simulink model "sgm_iox_io397_digital_loopback"  (R2020b)
settings: Solver=FixedStepDiscrete  StartTime=0.0  StopTime=inf  FixedStep=0.001  RelTol=1e-3  EnableMultiTasking=on
undefined symbols (not defined in the file): IO397
libraries: speedgoatlib_fpga_dio x2, speedgoatlib_fpga x1
settings Model: SimulationMode=external  ExtModeArmWhenConnect=off  Creator=ylee  LastModifiedBy=daniel.fonte
settings SolverCC: ConcurrentTasks=on  PositivePriorityOrder=on  AutoInsertRateTranBlk=on  InsertRTBMode=Never (minimum delay)
settings DataIOCC: SaveFormat=Array  SignalLoggingSaveFormat=ModelDataLogs  SaveState=on
settings OptimizationCC: BlockReduction=off  OptimizeBlockIOStorage=off  BufferReuse=off  GlobalBufferReuse=off  ExpressionFolding=off  ExpressionDepthLimit=2147483647  LocalBlockOutputs=off  InitFltsAndDblsToZero=on  OptimizeDataStoreBuffers=off  BusAssignmentInplaceUpdate=off
settings DebuggingCC: UnderspecifiedInitializationDetection=Classic  MergeDetectMultiDrivingBlocksExec=none  SolverPrmCheckMsg=warning  FcnCallInpInsideContextMsg=warning  AllowSymbolicDim=off  StateNameClashWarn=warning  SFUnexpectedBacktrackingDiag=warning  SFNoUnconditionalDefaultTransitionDiag=warning  SFExecutionAtInitializationDiag=none  ArithmeticOperatorsInVariantConditions=warning
settings HardwareCC: ProdBitPerLong=64  ProdLongLongMode=on  ProdHWDeviceType=Intel->x86-64 (Linux 64)
settings ModelReferenceCC: PropagateSignalLabelsOutOfModel=off
settings SFSimCC: SimCustomHeaderCode="#include \"my_type.h\""  SimUseLocalCustomCode=off  SimParseCustomCode=off  CustomCodeUndefinedFunction=UseInterfaceOnly
settings RTWCC: Description=Simulink Real-Time  SystemTargetFile=slrealtime.tlc  TemplateMakefile=slrealtime_default_tmf  RTWUseLocalCustomCode=off  Toolchain=Simulink Real-Time Toolchain  BuildConfiguration=Faster Runs  CodeExecutionProfiling=on  TargetLang=C++
settings CodeAppCC: StateflowObjectComments=on
settings ConfigComp: CovMetricSettings=dw  CovSaveCumulativeToWorkspaceVar=on  CovSaveSingleToWorkspaceVar=on  CovExternalEMLEnable=off  CovSFcnEnable=off

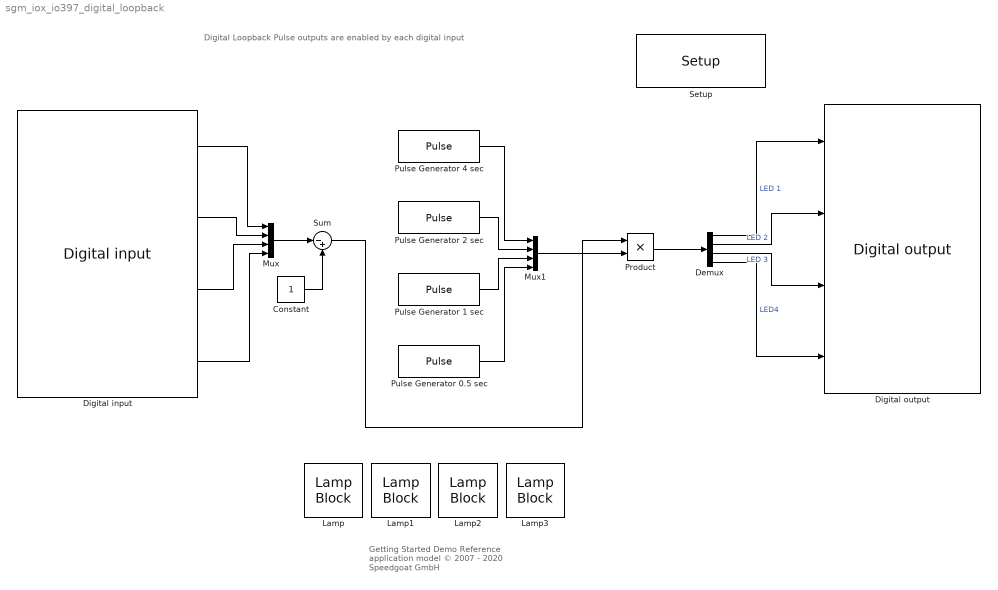
== system sgm_iox_io397_digital_loopback ==
  note: Digital Loopback
      | Pulse outputs are enabled by each digital input
  note: Getting Started Demo
      | Reference application model
      | © 2007 - 2020 Speedgoat GmbH
  Constant : Constant
  Demux : Demux
  Digital input : speedgoatlib_fpga_dio/Digital input  id=1  chan=[1 2 3 4]  ts=0.001  pciSlot=-1  board=IO397-50k  vectorizeOutput=off
      settings: SourceProductName=Simulink Real-Time: Speedgoat I/O Driver Library
  Digital output : speedgoatlib_fpga_dio/Digital output  id=1  chan=[5 6 7 8]  init=[0]  reset=[0]  vectorizeInput=off  ts=0.001  pciSlot=-1  board=IO397-50k
      settings: SourceProductName=Simulink Real-Time: Speedgoat I/O Driver Library
  Lamp{,1..3} (4 alike) : LampBlock
  Mux : Mux
  Mux1 : Mux
  Product : Product
  Pulse Generator 0.5 sec : DiscretePulseGenerator  PulseType=Time based  Period=0.5  PulseWidth=50
  Pulse Generator 1 sec : DiscretePulseGenerator  PulseType=Time based  Period=1  PulseWidth=50
  Pulse Generator 2 sec : DiscretePulseGenerator  PulseType=Time based  PulseWidth=50
  Pulse Generator 4 sec : DiscretePulseGenerator  PulseType=Time based  Period=4  PulseWidth=50
  Setup : speedgoatlib_fpga/Setup/Setup  board=IO397-50k  id=1  device_id=1  frontIO=None  rearIO=None  bitstreamFile=speedgoat_IO397_50k_CI_IO397_DUT_DEMO  rev=1.0  timestamp_string=05/10/17 09:15:16  fpgaFreq=75 MHz  fpgaTick=13.33 ns  ProgSpiFlash=off  ProgBPIFlash=off  pciSlot=-1  PullRPort0=pull-up 3.3V  VioPort0=3.3V  PullRPort1=pull-up 3.3V  VioPort1=3.3V  PullRPort2=pull-up 3.3V  VioPort2=3.3V  PullRPort3=pull-up 3.3V  VioPort3=3.3V  PullRPort4=pull-up 3.3V  VioPort4=3.3V  PullRPort5=pull-up 3.3V  VioPort5=3.3V  PullRPort6=pull-up 3.3V  VioPort6=3.3V  PullRPort15=pull-up 3.3V  PullRPort31=pull-up 3.3V  PullRPort47=pull-up 3.3V  PullRPort63=pull-up 3.3V
      settings: SourceProductName=Simulink Real-Time: Speedgoat I/O Driver Library
  Sum : Sum  Inputs=|-+
  wires:
  Digital input/2 -> Mux/2
  Digital input/3 -> Mux/3
  Digital input/1 -> Mux/1
  Digital input/4 -> Mux/4
  Pulse Generator 2 sec/1 -> Mux1/2
  Pulse Generator 1 sec/1 -> Mux1/3
  Pulse Generator 4 sec/1 -> Mux1/1
  Pulse Generator 0.5 sec/1 -> Mux1/4
  Mux/1 -> Sum/1
  Constant/1 -> Sum/2
  Sum/1 -> Product/1
  Mux1/1 -> Product/2
  Product/1 -> Demux/1
  Demux/2 -> Digital output/2  "LED 2"
  Demux/3 -> Digital output/3  "LED 3"
  Demux/1 -> Digital output/1  "LED 1"
  Demux/4 -> Digital output/4  "LED4"
